simulink model "pendule_inv_capteur_etu"  (R2021a)
settings: Solver=VariableStepAuto  StartTime=0.0  StopTime=10.0  RelTol=1e-3
undefined symbols (not defined in the file): g, K, l, ue, x0, xe
settings Model: Creator=ftestu  LastModifiedBy=ftestu

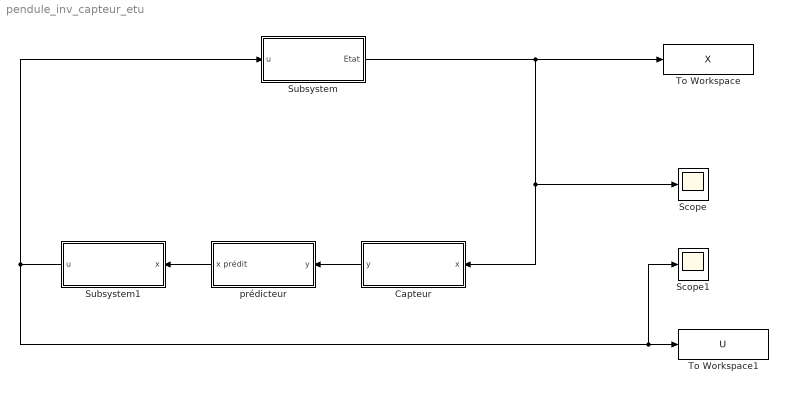
== system pendule_inv_capteur_etu ==
  Capteur : Subsystem
  Scope : Scope
  Scope1 : Scope
  Subsystem : Subsystem
  Subsystem1 : Subsystem
  To Workspace : ToWorkspace  VariableName=X  SaveFormat=Timeseries  SampleTime=-1
  To Workspace1 : ToWorkspace  VariableName=U  SaveFormat=Timeseries  SampleTime=-1
  prédicteur : Subsystem
  wires:
  Subsystem1/1(u) -> Scope1/1, To Workspace1/1, Subsystem/1(u)
  Subsystem/1(Etat) -> Capteur/1(x), Scope/1, To Workspace/1
  Capteur/1(y) -> prédicteur/1(y)
  prédicteur/1(x prédit) -> Subsystem1/1(x)

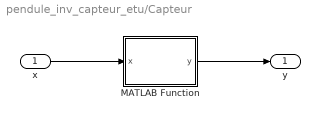
== system pendule_inv_capteur_etu/Capteur ==
  x : Inport
  MATLAB Function : MATLAB Function  TreatAsAtomicUnit=on
  y : Outport
  wires:
  x/1 -> MATLAB Function/1(x)
  MATLAB Function/1(y) -> y/1

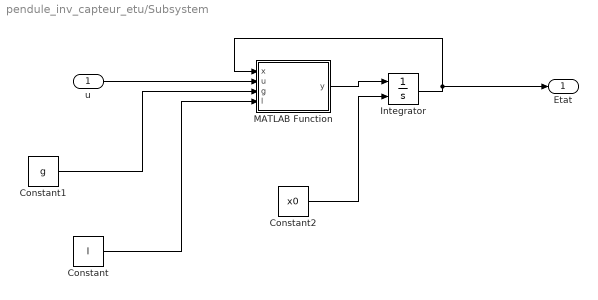
== system pendule_inv_capteur_etu/Subsystem ==
  u : Inport
  Constant : Constant  Value=l
  Constant1 : Constant  Value=g
  Constant2 : Constant  Value=x0
  Integrator : Integrator  InitialConditionSource=external
  MATLAB Function : MATLAB Function  TreatAsAtomicUnit=on
  Etat : Outport
  wires:
  u/1 -> MATLAB Function/2(u)
  Constant/1 -> MATLAB Function/4(l)
  Constant1/1 -> MATLAB Function/3(g)
  MATLAB Function/1(y) -> Integrator/1
  Integrator/1 -> Etat/1, MATLAB Function/1(x)
  Constant2/1 -> Integrator/2

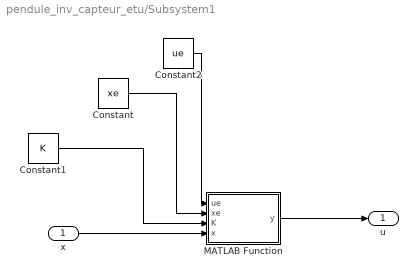
== system pendule_inv_capteur_etu/Subsystem1 ==
  x : Inport
  Constant : Constant  Value=xe
  Constant1 : Constant  Value=K
  Constant2 : Constant  Value=ue
  MATLAB Function : MATLAB Function  TreatAsAtomicUnit=on
  u : Outport
  wires:
  x/1 -> MATLAB Function/4(x)
  Constant1/1 -> MATLAB Function/3(K)
  Constant/1 -> MATLAB Function/2(xe)
  Constant2/1 -> MATLAB Function/1(ue)
  MATLAB Function/1(y) -> u/1

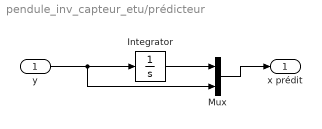
== system pendule_inv_capteur_etu/prédicteur ==
  y : Inport
  Integrator : Integrator
  Mux : Mux  Inputs=2
  x prédit : Outport
  wires:
  y/1 -> Mux/2, Integrator/1
  Integrator/1 -> Mux/1
  Mux/1 -> x prédit/1

== matlab function pendule_inv_capteur_etu/Subsystem1/MATLAB Function ==
  data: ue input; xe input; K input; x input; y output
function y = fcn(ue,xe,K,x)
y = ue+K(1)*(x(1)-xe(1)) + K(2)*(x(2)-xe(2));
end

== matlab function pendule_inv_capteur_etu/Subsystem/MATLAB Function ==
  data: x input; u input; y output; g input; l input
function y = fcn(x,u,g,l)
y = [x(2), g/l*sin(x(1))-u*cos(x(1))/l]';
end

== matlab function pendule_inv_capteur_etu/Capteur/MATLAB Function ==
  data: x input; y output
function y = fcn(x)

y = x(2);
